simulink model "ManeuverPlanning"  (R2020b)
settings: Solver=FixedStepAuto  StartTime=0.0  StopTime=15  FixedStep=Ts/2  RelTol=1e-3
values from neighbouring files (symbols this model uses):
  Ts = 0.01    [prepare_simulation.m]
undefined symbols (not defined in the file or in its folder): constraints, dimensionsEgo, dimensionsLead, ego, laneWidth, lateral, other, road, roadTrajectory, uncertainty, v_max, v_min, wheelBaseEgo, wheelBaseLead, xEgo_0, yawEgo_0, yEgo_0
libraries: sim3dautolib x3, mpcadaslib x2, vrlib x2, simulink x2, robotalgslib x1, drivingvehiclecontroller x1, pid_lib x1, sim3dlib x1, robotmobilelib x1
(part 1 of 2)
settings Model: Creator=Mustafa  LastModifiedBy=mustafa
settings SFSimCC: CustomCodeUndefinedFunction=UseInterfaceOnly

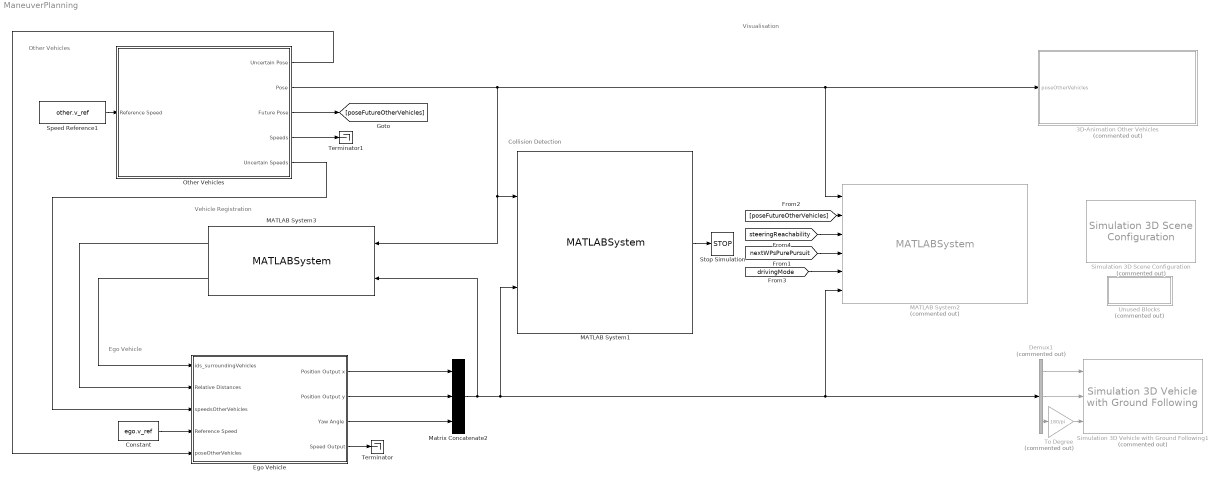
== system ManeuverPlanning ==
  note: Vehicle Registration
  note: Collision Detection
  note: Visualisation
  note: Ego Vehicle
  note: Other Vehicles
  3D-Animation Other Vehicles : Subsystem  Commented=on
  Constant : Constant  Value=ego.v_ref
  Demux1 : Demux  Commented=on  Outputs=3
  Ego Vehicle : Subsystem  mask{Speed=ego.v_0}
      mask prompts: Speed "Initial Speed"
      mask TypeOptions Speed: Initial Speed/Value
  MATLAB System1 : MATLABSystem  System=CollisionDetection  dimensionsEgo=ego.dimensions  wheelBaseEgo=ego.wheelBase  dimensionsOtherVehicles=other.dimensions  wheelBaseOtherVehicles=other.wheelBase  SimulateUsing=Interpreted execution
      mask Type: CollisionDetection
      mask Display:
      | disp('CollisionDetection');
      | port_label('input',1,'poseOtherVehicles');
      | port_label('input',2,'poseEgo');
      | port_label('output',1,'isCollided');
  MATLAB System2 : MATLABSystem  Commented=on  System=PlotDrivingScenario  dimensionsOtherVehicles=other.dimensions  wheelBaseOtherVehicles=other.wheelBase  dimensionsEgo=ego.dimensions  wheelBaseEgo=ego.wheelBase  LaneWidth=road.laneWidth  RoadTrajectory=road.trajectory  spaceDiscretisation=spaceDiscretisation  SimulateUsing=Interpreted execution
      mask Type: PlotDrivingScenario
      mask Display:
      | disp('PlotDrivingScenario');
      | port_label('input',1,'poseOtherVehicles');
      | port_label('input',2,'poseOtherVehiclesFuture');
      | port_label('input',3,'egoReachability');
      | port_label('input',4,'nextWPsPurePursuit');
      | port_label('input',5,'currentDrivingMode');
      | port_label('input',6,'poseEgo');
  MATLAB System3 : MATLABSystem  System=RegisterVehicles  LaneWidth=road.laneWidth  RoadTrajectory=road.trajectory  SimulateUsing=Interpreted execution
      mask Type: RegisterVehicles
      mask Display:
      | disp('RegisterVehicles');
      | port_label('input',1,'poseOtherVehicles');
      | port_label('input',2,'poseEgo');
      | port_label('output',1,'distances2Vehicles');
      | port_label('output',2,'ids_surroundingVehicles');
  Matrix Concatenate2 : Concatenate  NumInputs=3  ConcatenateDimension=2
  Other Vehicles : Subsystem  mask{s_0=other.s_0, d=other.d_0, Speed=other.v_0}
      mask prompts: s_0 "Initial s (Frenet)"; d "d (Frenet)"; Speed "Initial Speed"
      mask TypeOptions s_0: Initial Frenet s-coordinate/Value
      mask TypeOptions d: Frenet d-coordinate/Value
      mask TypeOptions Speed: Initial Speed/Value
  Simulation 3D Scene Configuration : sim3dlib/Simulation 3D Scene Configuration  Priority=0  Commented=on  ProjectFormat=Default Scenes  SceneDesc=Straight road  ProjectName=VehicleSimulation.exe  ScenePath=/Game/Maps/HwStrght  vehTagList={'Scene Origin';'SimulinkVehicle1';'SimulinkVehicle2';'SimulinkVehicleEgo'}  vehTag=SimulinkVehicleEgo  OpVisEn=off  Ts=0.1  EnableWindow=on  sensorTag=MainCamera1  sensorId=1  sensorName=MainCamera1  mountLoc=Origin  offsetFlag=off  tmountOffset=[0, 0, 0]  rmountOffset=[0, 0, 0]  HorizontalResolution=1280  VerticalResolution=720  HorizontalFOV=60  mountPoint=[0 0 0]  mountOrientation=[0 0 0]  aMode=3  ID=1
      settings: SourceProductBaseCode=DR,UV,VE
  Simulation 3D Vehicle with Ground Following1 : sim3dautolib/Simulation 3D Vehicle with Ground Following  Priority=-1  Commented=on  PassVehMesh=Muscle car  VehColor=Red  InitialPos=[ego.x_0, ego.y_0, ego.yaw_0]  InitialRot=[0, 0, 0]  ActorName=SimulinkVehicleEgo  SampleTime=0.1  ActorType=SimulinkVehicle  ID=C  aMode=3  ActorTag=SimulinkVehicleEgo  CoordinateScheme=ISO  TransformOutportEnabled=off
      settings: SourceProductBaseCode=DR,UV,VE
  Speed Reference1 : Constant  Value=other.v_ref
  Stop Simulation : Stop
  Terminator : Terminator
  Terminator1 : Terminator
  To Degree : Gain  Commented=on  Gain=180/pi
  Unused Blocks : Subsystem  Commented=on
  wires:
  Ego Vehicle/1(Position Output x) -> Matrix Concatenate2/1
  Ego Vehicle/4(Speed Output) -> Terminator/1
  Ego Vehicle/2(Position Output y) -> Matrix Concatenate2/2
  Ego Vehicle/3(Yaw Angle) -> Matrix Concatenate2/3
  Matrix Concatenate2/1 -> MATLAB System3/2, MATLAB System1/2, MATLAB System2/6, Demux1/1
  Demux1/1 -> Simulation 3D Vehicle with Ground Following1/1
  Demux1/2 -> Simulation 3D Vehicle with Ground Following1/2
  Demux1/3 -> To Degree/1
  To Degree/1 -> Simulation 3D Vehicle with Ground Following1/3
  MATLAB System1/1 -> Stop Simulation/1
  Other Vehicles/2(Pose) -> MATLAB System1/1, MATLAB System3/1, MATLAB System2/1, 3D-Animation Other Vehicles/1(poseOtherVehicles)
  Constant/1 -> Ego Vehicle/4(Reference Speed)
  MATLAB System3/2 -> Ego Vehicle/1(ids_surroundingVehicles)
  MATLAB System3/1 -> Ego Vehicle/2(Relative Distances)
  [poseFutureOtherVehicles] -> MATLAB System2/2
  Other Vehicles/3(Future Pose) -> [poseFutureOtherVehicles]
  [steeringReachability] -> MATLAB System2/3
  [nextWPsPurePursuit] -> MATLAB System2/4
  [drivingMode] -> MATLAB System2/5
  Speed Reference1/1 -> Other Vehicles/1(Reference Speed)
  Other Vehicles/1(Uncertain Pose) -> Ego Vehicle/5(poseOtherVehicles)
  Other Vehicles/5(Uncertain Speeds) -> Ego Vehicle/3(speedsOtherVehicles)
  Other Vehicles/4(Speeds) -> Terminator1/1

== system ManeuverPlanning/3D-Animation Other Vehicles ==
  poseOtherVehicles : Inport
  Demux : Demux  Outputs=3
  Demux1 : Demux  Outputs=3
  Selector : Selector  NumberOfDimensions=2  InputPortWidth=3  IndexOptions=Select all,Index vector (dialog)  Indices=[1 3],1  OutputSizes=1,1
  Selector1 : Selector  NumberOfDimensions=2  InputPortWidth=3  IndexOptions=Select all,Index vector (dialog)  Indices=[1 3],2  OutputSizes=1,1
  Simulation 3D Vehicle with Ground Following : sim3dautolib/Simulation 3D Vehicle with Ground Following  Priority=-1  PassVehMesh=Small pickup truck  VehColor=Blue  InitialPos=[other.x_0(1), other.y_0(1), other.yaw_0(1)]  InitialRot=[0, 0, 0]  ActorName=SimulinkVehicle1  SampleTime=0.1  ActorType=SimulinkVehicle  ID=1  aMode=3  ActorTag=SimulinkVehicle1  CoordinateScheme=ISO  TransformOutportEnabled=off
      settings: SourceProductBaseCode=DR,UV,VE
  Simulation 3D Vehicle with Ground Following1 : sim3dautolib/Simulation 3D Vehicle with Ground Following  Priority=-1  PassVehMesh=Sedan  VehColor=Blue  InitialPos=[other.x_0(2), other.y_0(2), other.yaw_0(2)]  InitialRot=[0, 0, 0]  ActorName=SimulinkVehicle2  SampleTime=0.1  ActorType=SimulinkVehicle  ID=2  aMode=3  ActorTag=SimulinkVehicle2  CoordinateScheme=ISO  TransformOutportEnabled=off
      settings: SourceProductBaseCode=DR,UV,VE
  To Degree1 : Gain  Gain=180/pi
  To Degree2 : Gain  Gain=180/pi
  wires:
  Demux/2 -> Simulation 3D Vehicle with Ground Following/2
  Demux/1 -> Simulation 3D Vehicle with Ground Following/1
  Demux/3 -> To Degree1/1
  To Degree1/1 -> Simulation 3D Vehicle with Ground Following/3
  To Degree2/1 -> Simulation 3D Vehicle with Ground Following1/3
  Demux1/1 -> Simulation 3D Vehicle with Ground Following1/1
  Demux1/3 -> To Degree2/1
  Demux1/2 -> Simulation 3D Vehicle with Ground Following1/2
  poseOtherVehicles/1 -> Selector/1, Selector1/1
  Selector/1 -> Demux/1
  Selector1/1 -> Demux1/1

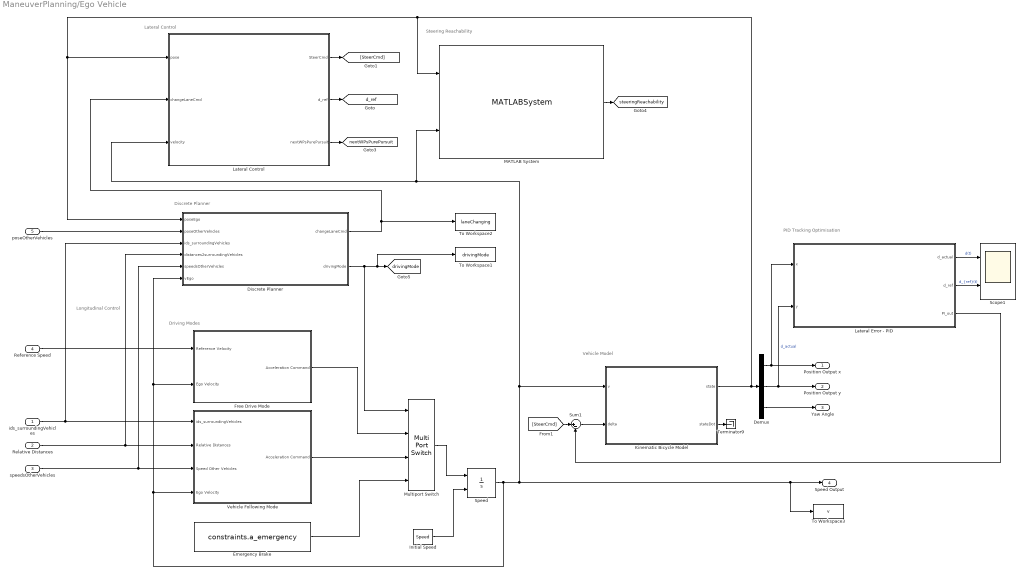
== system ManeuverPlanning/Ego Vehicle ==
  note: PID Tracking Optimisation
  note: Vehicle Model
  note: Discrete Planner
  note: Driving Modes
  note: Longitudinal Control
  note: Lateral Control
  note: Steering Reachability
  ids_surroundingVehicles : Inport
  Relative Distances : Inport  Port=2
  speedsOtherVehicles : Inport  Port=3
  Reference Speed : Inport  Port=4
  poseOtherVehicles : Inport  Port=5
  Demux : Demux  Outputs=3
  Discrete Planner : Subsystem  Variant=on  VariantControlMode=label  LabelModeActiveChoice=POMDP  mask{modePlanner=POMDP}
      mask prompts: modePlanner "Planner Mode:"
      mask TypeOptions modePlanner: MANUAL | FORMAL | NEWPLANNER | POMDP
      mask Callback modePlanner: set_param(gcb,'OverrideUsingVariant',get_param(gcb,'modePlanner'));
  Emergency Brake : Constant  Value=constraints.a_emergency
  Free Drive Mode : Subsystem
  Initial Speed : Constant  Value=Speed
  Kinematic Bicycle Model : Subsystem  mask{L=ego.wheelBase, v_min=constraints.v_min, v_max=constraints.v_max, delta_min=-constraints.steerAngle_max, delta_max=constraints.steerAngle_max, x_0=ego.x_0, y_0=ego.y_0, theta_0=ego.yaw_0}
      mask prompts: L "Wheel base (m):"; v_min "Minimum velocity (m/s):"; v_max "Maximum velocity (m/s):"; delta_min "Minimum steering angle (rad):"; delta_max "Maximum steering angle (rad):"; x_0 "Initial x (m):"; y_0 "Initial y (m):"; theta_0 "Initial orientation (rad):"
      mask TypeOptions L: wheel base/Value
      mask TypeOptions v_min: limit velocity/LowerLimit
      mask TypeOptions v_max: limit velocity/UpperLimit
      mask TypeOptions delta_min: limit steering angle/LowerLimit
      mask TypeOptions delta_max: limit steering angle/UpperLimit
      mask TypeOptions x_0: x_0/Value
      mask TypeOptions y_0: y_0/Value
      mask TypeOptions theta_0: theta_0/Value
  Lateral Control : Subsystem  Variant=on  VariantControlMode=label  LabelModeActiveChoice=STANLEY  mask{modeLateral=STANLEY}
      mask prompts: modeLateral "Lateral Mode:"
      mask TypeOptions modeLateral: PURE_PURSUIT | STANLEY
      mask Callback modeLateral: set_param(gcb,'OverrideUsingVariant',get_param(gcb,'modeLateral'))
  Lateral Error - PID : Subsystem
  MATLAB System : MATLABSystem  System=SteeringReachability  minimumAcceleration=constraints.a_min  maximumAcceleration=constraints.a_max  emergencyAcceleration=constraints.a_emergency  maximumVelocity=constraints.v_max  RoadTrajectory=road.trajectory  wheelBase=ego.wheelBase  steerAngle_max=constraints.steerAngle_max  timeHorizon=trajectoryGeneration.timeHorizon  Ts=Ts  SimulateUsing=Interpreted execution
      mask Type: SteeringReachability
      mask Display:
      | disp('SteeringReachability');
      | port_label('input',1,'pose');
      | port_label('input',2,'v');
      | port_label('output',1,'steeringReachability');
  Multiport Switch : MultiPortSwitch
  Scope1 : Scope  NumInputPorts=2
  Speed : Integrator  InitialConditionSource=external  LimitOutput=on  UpperSaturationLimit=constraints.v_max  LowerSaturationLimit=constraints.v_min
  Sum1 : Sum  Inputs=|+-
  Terminator9 : Terminator
  To Workspace1 : ToWorkspace  VariableName=drivingMode  SampleTime=-1
      settings: Save2DSignal=2-D array (concatenate along first dimension)
  To Workspace2 : ToWorkspace  VariableName=laneChanging  SampleTime=-1
      settings: Save2DSignal=2-D array (concatenate along first dimension)
  To Workspace3 : ToWorkspace  VariableName=v  SampleTime=-1
      settings: Save2DSignal=2-D array (concatenate along first dimension)
  Vehicle Following Mode : Subsystem
  Position Output x : Outport  VectorParamsAs1DForOutWhenUnconnected=off
  Position Output y : Outport  Port=2  VectorParamsAs1DForOutWhenUnconnected=off
  Yaw Angle : Outport  Port=3  VectorParamsAs1DForOutWhenUnconnected=off
  Speed Output : Outport  Port=4  VectorParamsAs1DForOutWhenUnconnected=off
  tag scope: d_ref=global, drivingMode=global, nextWPsPurePursuit=global, steeringReachability=global
  wires:
  Initial Speed/1 -> Speed/2
  Vehicle Following Mode/1(Acceleration Command) -> Multiport Switch/3
  Multiport Switch/1 -> Speed/1
  Free Drive Mode/1(Acceleration Command) -> Multiport Switch/2
  Emergency Brake/1 -> Multiport Switch/4
  Demux/3 -> Yaw Angle/1
  Kinematic Bicycle Model/2(stateDot) -> Terminator9/1
  Demux/2 -> Position Output y/1, Lateral Error - PID/2(y)  "d_actual"
  Lateral Control/1(SteerCmd) -> [SteerCmd]
  Lateral Control/2(d_ref) -> [d_ref]
  Discrete Planner/1(changeLaneCmd) -> Lateral Control/2(changeLaneCmd), To Workspace2/1
  Speed/1 -> To Workspace3/1, Speed Output/1, Kinematic Bicycle Model/1(v), MATLAB System/2, Lateral Control/3(velocity), Vehicle Following Mode/4(Ego Velocity), Discrete Planner/6(vEgo), Free Drive Mode/2(Ego Velocity)
  Kinematic Bicycle Model/1(state) -> MATLAB System/1, Discrete Planner/1(poseEgo), Lateral Control/1(pose), Demux/1
  Lateral Control/3(nextWPsPurePursuit) -> [nextWPsPurePursuit]
  Sum1/1 -> Kinematic Bicycle Model/2(delta)
  [SteerCmd] -> Sum1/1
  Lateral Error - PID/3(PI_out) -> Sum1/2
  Demux/1 -> Position Output x/1, Lateral Error - PID/1(x)
  Lateral Error - PID/1(d_actual) -> Scope1/1  "d(t)"
  Lateral Error - PID/2(d_ref) -> Scope1/2  "d_{ref}(t)"
  Reference Speed/1 -> Free Drive Mode/1(Reference Velocity)
  Relative Distances/1 -> Discrete Planner/4(distances2surroundingVehicles), Vehicle Following Mode/2(Relative Distances)
  speedsOtherVehicles/1 -> Discrete Planner/5(speedsOtherVehicles), Vehicle Following Mode/3(Speed Other Vehicles)
  Discrete Planner/2(drivingMode) -> Multiport Switch/1, To Workspace1/1, [drivingMode]
  ids_surroundingVehicles/1 -> Discrete Planner/3(ids_surroundingVehicles), Vehicle Following Mode/1(ids_surroundingVehicles)
  MATLAB System/1 -> [steeringReachability]
  poseOtherVehicles/1 -> Discrete Planner/2(poseOtherVehicles)

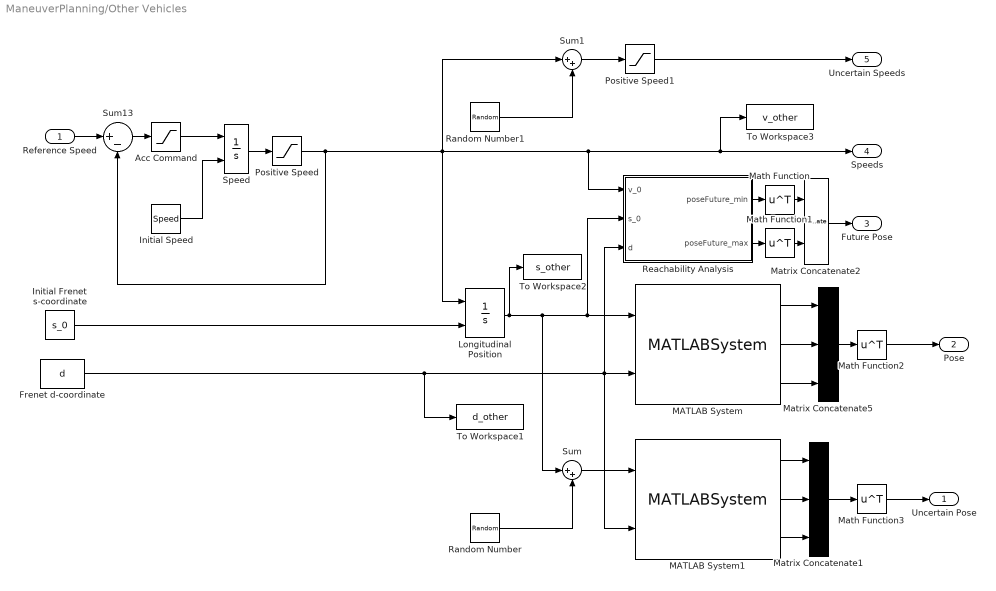
== system ManeuverPlanning/Other Vehicles ==
  Reference Speed : Inport
  Acc Command : Saturate  UpperLimit=constraints.a_max  LowerLimit=constraints.a_min
  Frenet d-coordinate : Constant  Value=d
  Initial Frenet s-coordinate : Constant  Value=s_0
  Initial Speed : Constant  Value=Speed
  Longitudinal Position : Integrator  InitialConditionSource=external
  MATLAB System : MATLABSystem  System=Frenet2CartesianSystem  RoadTrajectory=road.trajectory  lengthOut=other.number  SimulateUsing=Interpreted execution
      mask Type: Frenet2CartesianSystem
      mask Display:
      | disp('Frenet2CartesianSystem');
      | port_label('input',1,'s');
      | port_label('input',2,'d');
      | port_label('output',1,'x');
      | port_label('output',2,'y');
      | port_label('output',3,'refOrientation');
  MATLAB System1 : MATLABSystem  System=Frenet2CartesianSystem  RoadTrajectory=road.trajectory  lengthOut=other.number  SimulateUsing=Interpreted execution
      mask Type: Frenet2CartesianSystem
      mask Display:
      | disp('Frenet2CartesianSystem');
      | port_label('input',1,'s');
      | port_label('input',2,'d');
      | port_label('output',1,'x');
      | port_label('output',2,'y');
      | port_label('output',3,'refOrientation');
  Math Function{,1..3} (4 alike) : Math  Operator=transpose  SaturateOnIntegerOverflow=on
  Matrix Concatenate1 : Concatenate  NumInputs=3  Mode=Multidimensional array  ConcatenateDimension=2
  Matrix Concatenate2 : Concatenate  Mode=Multidimensional array
  Matrix Concatenate5 : Concatenate  NumInputs=3  Mode=Multidimensional array  ConcatenateDimension=2
  Positive Speed : Saturate  UpperLimit=constraints.v_max  LowerLimit=constraints.v_min
  Positive Speed1 : Saturate  UpperLimit=constraints.v_max  LowerLimit=constraints.v_min
  Random Number : RandomNumber  Variance=uncertainty.sigmaS^2  SampleTime=Ts
  Random Number1 : RandomNumber  Variance=uncertainty.sigmaV^2  SampleTime=Ts
  Reachability Analysis : Subsystem
  Speed : Integrator  InitialConditionSource=external
  Sum : Sum  Inputs=|++
  Sum1 : Sum  Inputs=|++
  Sum13 : Sum  Inputs=|+-
  To Workspace1 : ToWorkspace  VariableName=d_other  SampleTime=-1
      settings: Save2DSignal=2-D array (concatenate along first dimension)
  To Workspace2 : ToWorkspace  VariableName=s_other  SampleTime=-1
      settings: Save2DSignal=2-D array (concatenate along first dimension)
  To Workspace3 : ToWorkspace  VariableName=v_other  SampleTime=-1
      settings: Save2DSignal=2-D array (concatenate along first dimension)
  Uncertain Pose : Outport  VectorParamsAs1DForOutWhenUnconnected=off
  Pose : Outport  Port=2
  Future Pose : Outport  Port=3
  Speeds : Outport  Port=4  VectorParamsAs1DForOutWhenUnconnected=off
  Uncertain Speeds : Outport  Port=5  VectorParamsAs1DForOutWhenUnconnected=off
  wires:
  Speed/1 -> Positive Speed/1
  Initial Frenet s-coordinate/1 -> Longitudinal Position/2
  Sum13/1 -> Acc Command/1
  Reference Speed/1 -> Sum13/1
  Acc Command/1 -> Speed/1
  Initial Speed/1 -> Speed/2
  Frenet d-coordinate/1 -> To Workspace1/1, MATLAB System1/2, MATLAB System/2, Reachability Analysis/3(d)
  Longitudinal Position/1 -> Sum/1, MATLAB System/1, Reachability Analysis/2(s_0), To Workspace2/1
  Matrix Concatenate2/1 -> Future Pose/1
  Reachability Analysis/1(poseFuture_min) -> Math Function/1
  Math Function/1 -> Matrix Concatenate2/1
  Reachability Analysis/2(poseFuture_max) -> Math Function1/1
  Math Function1/1 -> Matrix Concatenate2/2
  Matrix Concatenate5/1 -> Math Function2/1
  MATLAB System/2 -> Matrix Concatenate5/2
  MATLAB System/1 -> Matrix Concatenate5/1
  MATLAB System/3 -> Matrix Concatenate5/3
  Math Function2/1 -> Pose/1
  Math Function3/1 -> Uncertain Pose/1
  Matrix Concatenate1/1 -> Math Function3/1
  MATLAB System1/3 -> Matrix Concatenate1/3
  MATLAB System1/2 -> Matrix Concatenate1/2
  MATLAB System1/1 -> Matrix Concatenate1/1
  Sum/1 -> MATLAB System1/1
  Random Number/1 -> Sum/2
  Random Number1/1 -> Sum1/2
  Sum1/1 -> Positive Speed1/1
  Positive Speed1/1 -> Uncertain Speeds/1
  Positive Speed/1 -> Sum1/1, To Workspace3/1, Speeds/1, Reachability Analysis/1(v_0), Longitudinal Position/1, Sum13/2

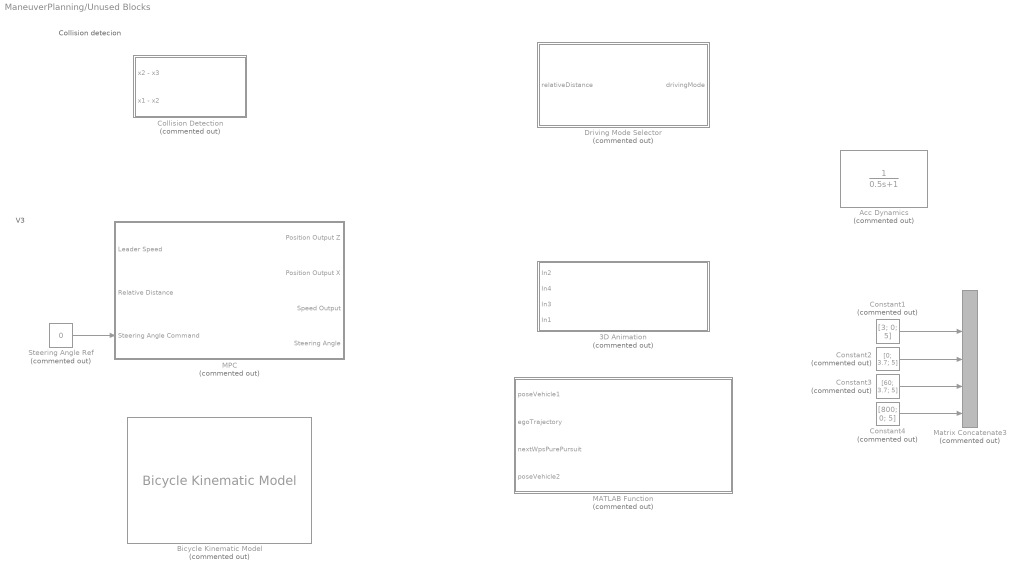
== system ManeuverPlanning/Unused Blocks ==
  note: V3
  note: Collision detecion
  3D Animation : Subsystem  Commented=on
  Acc Dynamics : TransferFcn  Commented=on  Denominator=[0.5 1]
  Bicycle Kinematic Model : robotmobilelib/Bicycle Kinematic Model  Commented=on  VehicleInputs=Vehicle Speed & Steering Angle  WheelBase=wheelBaseEgo  VehicleSpeedRange=[v_min v_max]  MaxSteeringAngle=steerAngle_max  InitialState=[xEgo_0; yEgo_0; yawEgo_0]  SimulateUsing=Interpreted execution
      settings: SourceProductBaseCode=RO
  Collision Detection : Subsystem  Commented=on
  Constant1 : Constant  Commented=on  Value=[3; 0; 5]
  Constant2 : Constant  Commented=on  Value=[0; 3.7; 5]
  Constant3 : Constant  Commented=on  Value=[60; 3.7; 5]
  Constant4 : Constant  Commented=on  Value=[800; 0; 5]
  Driving Mode Selector : Stateflow chart  Commented=on  TreatAsAtomicUnit=on
  MATLAB Function : MATLAB Function  Commented=on  TreatAsAtomicUnit=on  SystemSampleTime=0.1  mask{dimensionsVehicle1=dimensionsLead, wheelBaseVehicle1=wheelBaseLead, dimensionsVehicle2=dimensionsEgo, wheelBaseVehicle2=wheelBaseEgo, LaneWidth=laneWidth, roadTrajectory=roadTrajectory}
      mask prompts: dimensionsVehicle1 "Dimensions (length, width) vehicle 1"; wheelBaseVehicle1 "Wheel base vehicle 1"; dimensionsVehicle2 "Dimensions (length, width) vehicle 2"; wheelBaseVehicle2 "Wheel base vehicle 2"; LaneWidth "Lane width"; roadTrajectory "Road trajectory according to MOBATSim map format"
      mask init:
      | close all;
      | figure('units','normalized','outerposition',[0 0 1 1]);
      | grid on
      | axis equal
      | hold on
  MPC : Subsystem  Commented=on  mask{Pos=20, Speed=25}
      mask prompts: Pos "Initial Position"; Speed "Initial Speed"
      mask TypeOptions Pos: Initial Position Z/Value
      mask TypeOptions Speed: Initial Speed/Value
  Matrix Concatenate3 : Concatenate  Commented=on  NumInputs=5  Mode=Multidimensional array  ConcatenateDimension=2
  Steering Angle Ref : Constant  Commented=on  Value=0
  wires:
  Steering Angle Ref/1 -> MPC/3(Steering Angle Command)
  Constant3/1 -> Matrix Concatenate3/4
  Constant4/1 -> Matrix Concatenate3/5
  Constant2/1 -> Matrix Concatenate3/3
  Constant1/1 -> Matrix Concatenate3/2

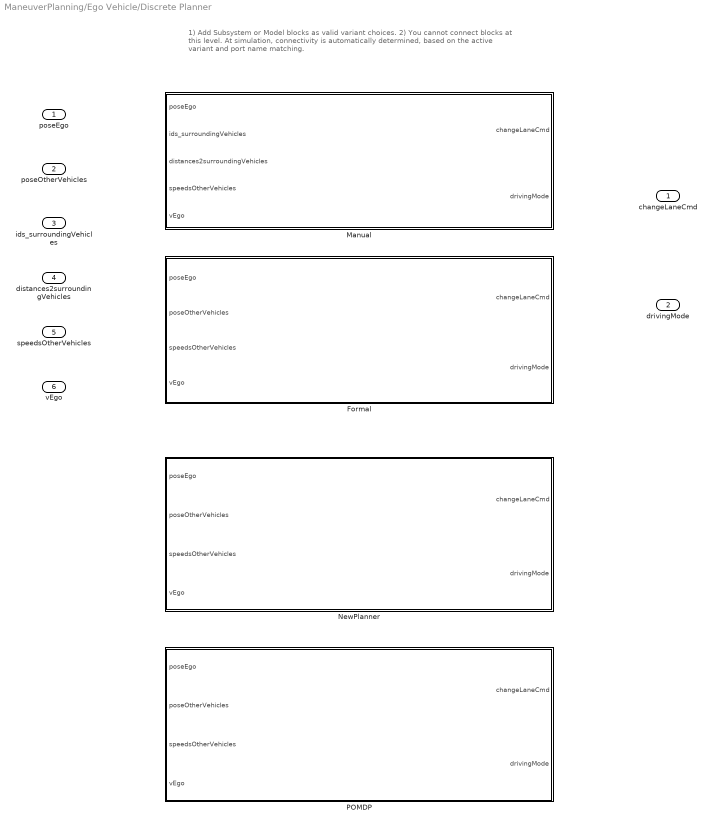
== system ManeuverPlanning/Ego Vehicle/Discrete Planner ==
  note: 1) Add Subsystem or Model blocks as valid variant choices.
      | 2) You cannot connect blocks at this level. At simulation, connectivity is automatically
      | determined, based on the active variant and port name matching.
  poseEgo : Inport
  poseOtherVehicles : Inport  Port=2
  ids_surroundingVehicles : Inport  Port=3
  distances2surroundingVehicles : Inport  Port=4
  speedsOtherVehicles : Inport  Port=5
  vEgo : Inport  Port=6
  Formal : Subsystem  VariantControl=FORMAL
  Manual : Subsystem  VariantControl=MANUAL
  NewPlanner : Subsystem  VariantControl=NEWPLANNER
  POMDP : Subsystem  VariantControl=POMDP
  changeLaneCmd : Outport
  drivingMode : Outport  Port=2

== system ManeuverPlanning/Ego Vehicle/Free Drive Mode ==
  Reference Velocity : Inport
  Ego Velocity : Inport  Port=2
  Acc Command : Saturate  UpperLimit=constraints.a_max  LowerLimit=constraints.a_min
  Sum13 : Sum  Inputs=|+-
  Acceleration Command : Outport
  wires:
  Sum13/1 -> Acc Command/1
  Acc Command/1 -> Acceleration Command/1
  Reference Velocity/1 -> Sum13/1
  Ego Velocity/1 -> Sum13/2

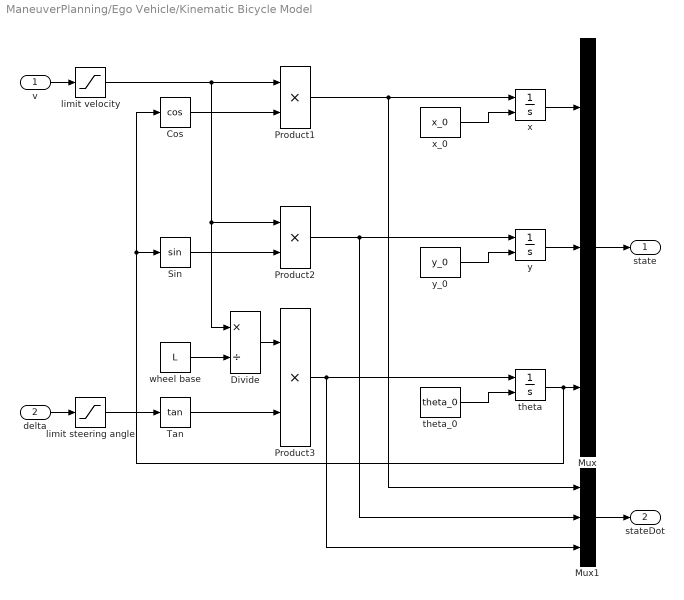
== system ManeuverPlanning/Ego Vehicle/Kinematic Bicycle Model ==
  v : Inport
  delta : Inport  Port=2
  Cos : Trigonometry  Operator=cos
  Divide : Product  Inputs=*/
  Mux : Mux  Inputs=3
  Mux1 : Mux  Inputs=3
  Product1 : Product
  Product2 : Product
  Product3 : Product
  Sin : Trigonometry
  Tan : Trigonometry  Operator=tan
  limit steering angle : Saturate  UpperLimit=delta_max  LowerLimit=delta_min
  limit velocity : Saturate  UpperLimit=v_max  LowerLimit=v_min
  theta : Integrator  InitialConditionSource=external
  theta_0 : Constant  Value=theta_0
  wheel base : Constant  Value=L
  x : Integrator  InitialConditionSource=external
  x_0 : Constant  Value=x_0
  y : Integrator  InitialConditionSource=external
  y_0 : Constant  Value=y_0
  state : Outport
  stateDot : Outport  Port=2
  wires:
  Mux/1 -> state/1
  Mux1/1 -> stateDot/1
  v/1 -> limit velocity/1
  Sin/1 -> Product2/2
  Cos/1 -> Product1/2
  Tan/1 -> Product3/2
  Product1/1 -> Mux1/1, x/1
  Product2/1 -> Mux1/2, y/1
  Product3/1 -> Mux1/3, theta/1
  theta/1 -> Cos/1, Sin/1, Mux/3
  x/1 -> Mux/1
  y/1 -> Mux/2
  Divide/1 -> Product3/1
  wheel base/1 -> Divide/2
  limit velocity/1 -> Product1/1, Divide/1, Product2/1
  x_0/1 -> x/2
  y_0/1 -> y/2
  theta_0/1 -> theta/2
  delta/1 -> limit steering angle/1
  limit steering angle/1 -> Tan/1

== system ManeuverPlanning/Ego Vehicle/Lateral Control ==
  note: 1) Add Subsystem or Model blocks as valid variant choices.
      | 2) You cannot connect blocks at this level. At simulation, connectivity is automatically
      | determined, based on the active variant and port name matching.
  pose : Inport
  changeLaneCmd : Inport  Port=2
  velocity : Inport  Port=3
  Pure Pursuit : Subsystem  VariantControl=PURE_PURSUIT
  Stanley : Subsystem  VariantControl=STANLEY
  SteerCmd : Outport
  d_ref : Outport  Port=2
  nextWPsPurePursuit : Outport  Port=3

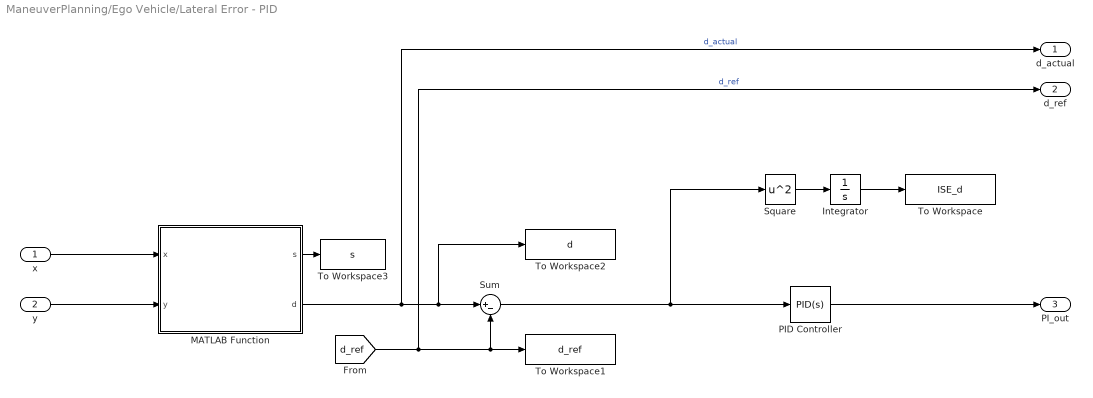
== system ManeuverPlanning/Ego Vehicle/Lateral Error - PID ==
  x : Inport
  y : Inport  Port=2
  Integrator : Integrator
  MATLAB Function : MATLAB Function  TreatAsAtomicUnit=on  mask{currentTrajectory=road.trajectory}
      mask prompts: currentTrajectory "Road trajectory"
  PID Controller : pid_lib/PID Controller  Controller=PID  Form=Parallel  TimeDomain=Continuous-time  UseExternalTs=off  SampleTime=-1  IntegratorMethod=Forward Euler  FilterMethod=Forward Euler  ControllerParametersSource=internal  P=lateral.Kp  I=lateral.Ki  D=lateral.Kd  UseFilter=on  N=100  TunerSelectOption=Transfer Function Based (PID Tuner App)  InitialConditionSource=internal  InitialConditionForIntegrator=0  InitialConditionForFilter=0  DifferentiatorICPrevScaledInput=0  ExternalReset=none  TrackingMode=off  Kt=1  LimitOutput=off  SatLimitsSource=internal  UpperSaturationLimit=inf  LowerSaturationLimit=-inf  LinearizeAsGain=on  AntiWindupMode=none  Kb=1  POutMin=[]  POutMax=[]  IOutMin=[]  IOutMax=[]  DOutMin=[]  DOutMax=[]  NOutMin=[]  NOutMax=[]  SumOutMin=[]  SumOutMax=[]  SaturationOutMin=[]  SaturationOutMax=[]  PParamMin=[]  PParamMax=[]  IParamMin=[]  IParamMax=[]  DParamMin=[]  DParamMax=[]  NParamMin=[]  NParamMax=[]  KbParamMin=[]  KbParamMax=[]  KtParamMin=[]  KtParamMax=[]  KbOutMin=[]  KbOutMax=[]  KtOutMin=[]  KtOutMax=[]  IntegratorOutMin=[]  IntegratorOutMax=[]  FilterOutMin=[]  FilterOutMax=[]  SumI1OutMin=[]  SumI1OutMax=[]  SumI2OutMin=[]  SumI2OutMax=[]  SumI3OutMin=[]  SumI3OutMax=[]  SumI4OutMin=[]  SumI4OutMax=[]  SumDOutMin=[]  SumDOutMax=[]  DifferentiatorOutMin=[]  DifferentiatorOutMax=[]  FilterDiffOutCoefMin=[]  FilterDiffOutCoefMax=[]  ReciprocalOutMin=[]  ReciprocalOutMax=[]  SumDenOutMin=[]  SumDenOutMax=[]  SumNumOutMin=[]  SumNumOutMax=[]  DivideOutMin=[]  DivideOutMax=[]  UdiffTsProdOutMin=[]  UdiffTsProdOutMax=[]  NTsProdOutMin=[]  NTsProdOutMax=[]  UintegralTsProdOutMin=[]  UintegralTsProdOutMax=[]  UngainTsProdOutMin=[]  UngainTsProdOutMax=[]  IntegratorContinuousStateAttributes=''  IntegratorStateMustResolveToSignalObject=off  IntegratorRTWStateStorageClass=Auto  FilterContinuousStateAttributes=''  FilterStateMustResolveToSignalObject=off  FilterRTWStateStorageClass=Auto  ParallelPVariant=InternalParameters  IdealPVariant=Disabled  IVariant=InternalParameters  DVariant=InternalParameters  IntegratorVariant=Continuous  SatVariant=Disabled  AWVariant=Passthrough  PCopyVariant=Disabled  TRVariant=Disabled  FdbkBlocksVariant=Forward  IdealPFdbkVariant=Disabled  SatFdbkVariant=Disabled  DerivativeFilterVariant=ContFilter  NVariant=InternalParameters  NCopyVariant=Disabled  FilterICVariant=InternalICsFilter  IntegratorICVariant=InternalICs  ExternalResetVariant=Disabled  TRSumVariant=Passthrough  SumFdbkVariant=Disabled  SumVariant=Sum_PID  TsampFilterVariant=InternalTs  TsampNgainVariant=Passthrough  TsampIntegralVariant=Passthrough  ExternalSaturationOutDataTypeStr=Inherit: Same as second input
  Square : Math  Operator=square  SaturateOnIntegerOverflow=on
  Sum : Sum  Inputs=|+-
  To Workspace : ToWorkspace  VariableName=ISE_d  SampleTime=-1
      settings: Save2DSignal=2-D array (concatenate along first dimension)
  To Workspace1 : ToWorkspace  VariableName=d_ref  SampleTime=-1
      settings: Save2DSignal=2-D array (concatenate along first dimension)
  To Workspace2 : ToWorkspace  VariableName=d  SampleTime=-1
      settings: Save2DSignal=2-D array (concatenate along first dimension)
  To Workspace3 : ToWorkspace  VariableName=s  SampleTime=-1
      settings: Save2DSignal=2-D array (concatenate along first dimension)
  d_actual : Outport
  d_ref : Outport  Port=2
  PI_out : Outport  Port=3
  wires:
  Sum/1 -> PID Controller/1, Square/1
  MATLAB Function/1(s) -> To Workspace3/1
  Integrator/1 -> To Workspace/1
  MATLAB Function/2(d) -> d_actual/1, To Workspace2/1, Sum/1  "d_actual"
  [d_ref] -> d_ref/1, To Workspace1/1, Sum/2  "d_ref"
  Square/1 -> Integrator/1
  y/1 -> MATLAB Function/2(y)
  x/1 -> MATLAB Function/1(x)
  PID Controller/1 -> PI_out/1

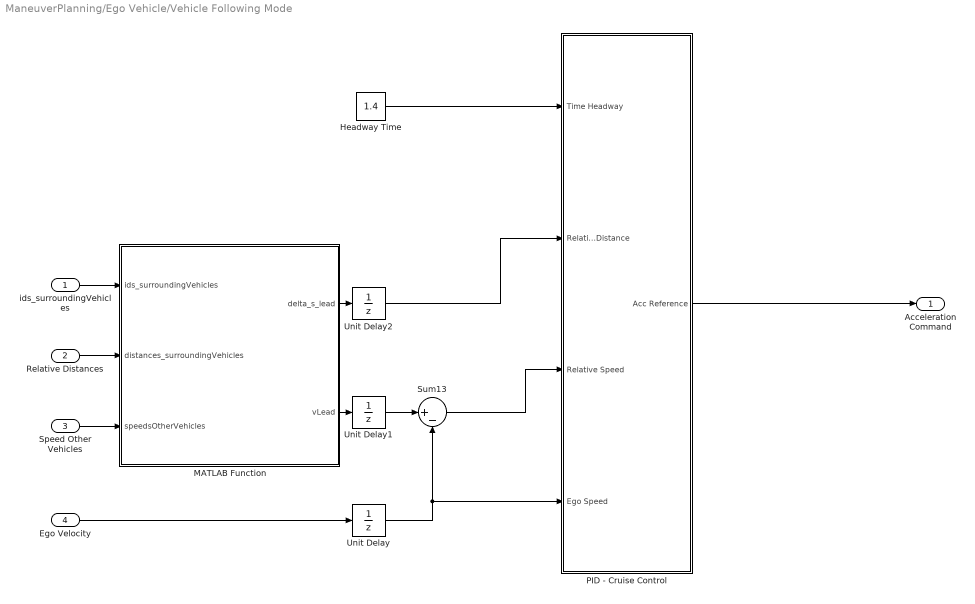
== system ManeuverPlanning/Ego Vehicle/Vehicle Following Mode ==
  ids_surroundingVehicles : Inport
  Relative Distances : Inport  Port=2
  Speed Other Vehicles : Inport  Port=3
  Ego Velocity : Inport  Port=4
  Headway Time : Constant  Value=1.4
  MATLAB Function : MATLAB Function  TreatAsAtomicUnit=on
  PID - Cruise Control : Subsystem
  Sum13 : Sum  Inputs=|+-
  Unit Delay : UnitDelay  SampleTime=-1  HasFrameUpgradeWarning=on
  Unit Delay1 : UnitDelay  SampleTime=-1  HasFrameUpgradeWarning=on
  Unit Delay2 : UnitDelay  SampleTime=-1  HasFrameUpgradeWarning=on
  Acceleration Command : Outport
  wires:
  Headway Time/1 -> PID - Cruise Control/1(Time Headway)
  Sum13/1 -> PID - Cruise Control/3(Relative Speed)
  PID - Cruise Control/1(Acc Reference) -> Acceleration Command/1
  Unit Delay/1 -> Sum13/2, PID - Cruise Control/4(Ego Speed)
  Unit Delay1/1 -> Sum13/1
  Unit Delay2/1 -> PID - Cruise Control/2(Relative Distance)
  MATLAB Function/1(delta_s_lead) -> Unit Delay2/1
  Ego Velocity/1 -> Unit Delay/1
  MATLAB Function/2(vLead) -> Unit Delay1/1
  Speed Other Vehicles/1 -> MATLAB Function/3(speedsOtherVehicles)
  ids_surroundingVehicles/1 -> MATLAB Function/1(ids_surroundingVehicles)
  Relative Distances/1 -> MATLAB Function/2(distances_surroundingVehicles)

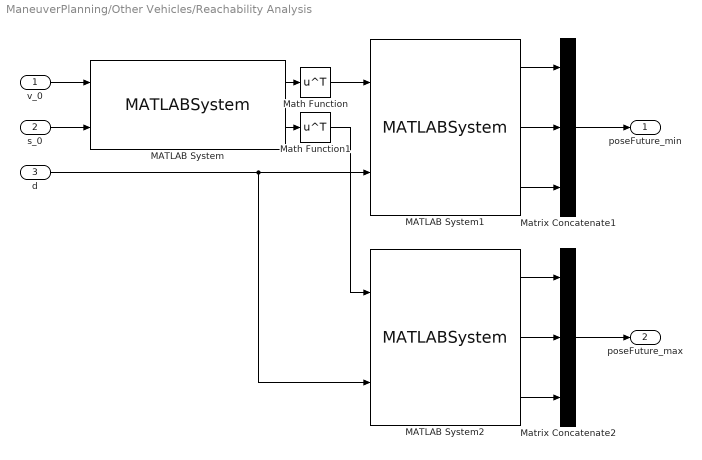
== system ManeuverPlanning/Other Vehicles/Reachability Analysis ==
  v_0 : Inport
  s_0 : Inport  Port=2
  d : Inport  Port=3
  MATLAB System : MATLABSystem  System=LongitudinalReachability  lengthOut=other.number  minimumAcceleration=constraints.a_min  maximumAcceleration=constraints.a_max  emergencyAcceleration=constraints.a_emergency  maximumVelocity=constraints.v_max  RoadTrajectory=road.trajectory  wheelBase=other.wheelBase(1)  steerAngle_max=constraints.steerAngle_max  timeHorizon=trajectoryGeneration.timeHorizon  Ts=Ts  SimulateUsing=Interpreted execution
      mask Type: LongitudinalReachability
      mask Display:
      | disp('LongitudinalReachability');
      | port_label('input',1,'v_0');
      | port_label('input',2,'s_0');
      | port_label('output',1,'sFuture_min');
      | port_label('output',2,'sFuture_max');
  MATLAB System1 : MATLABSystem  System=Frenet2CartesianSystem  RoadTrajectory=road.trajectory  lengthOut=other.number  SimulateUsing=Interpreted execution
      mask Type: Frenet2CartesianSystem
      mask Display:
      | disp('Frenet2CartesianSystem');
      | port_label('input',1,'s');
      | port_label('input',2,'d');
      | port_label('output',1,'x');
      | port_label('output',2,'y');
      | port_label('output',3,'refOrientation');
  MATLAB System2 : MATLABSystem  System=Frenet2CartesianSystem  RoadTrajectory=road.trajectory  lengthOut=other.number  SimulateUsing=Interpreted execution
      mask Type: Frenet2CartesianSystem
      mask Display:
      | disp('Frenet2CartesianSystem');
      | port_label('input',1,'s');
      | port_label('input',2,'d');
      | port_label('output',1,'x');
      | port_label('output',2,'y');
      | port_label('output',3,'refOrientation');
  Math Function : Math  Operator=transpose  SaturateOnIntegerOverflow=on
  Math Function1 : Math  Operator=transpose  SaturateOnIntegerOverflow=on
  Matrix Concatenate1 : Concatenate  NumInputs=3  Mode=Multidimensional array  ConcatenateDimension=2
  Matrix Concatenate2 : Concatenate  NumInputs=3  Mode=Multidimensional array  ConcatenateDimension=2
  poseFuture_min : Outport
  poseFuture_max : Outport  Port=2
  wires:
  s_0/1 -> MATLAB System/2
  v_0/1 -> MATLAB System/1
  d/1 -> MATLAB System2/2, MATLAB System1/2
  MATLAB System1/1 -> Matrix Concatenate1/1
  MATLAB System1/2 -> Matrix Concatenate1/2
  MATLAB System1/3 -> Matrix Concatenate1/3
  MATLAB System2/1 -> Matrix Concatenate2/1
  MATLAB System2/2 -> Matrix Concatenate2/2
  MATLAB System2/3 -> Matrix Concatenate2/3
  Matrix Concatenate1/1 -> poseFuture_min/1
  Matrix Concatenate2/1 -> poseFuture_max/1
  MATLAB System/2 -> Math Function1/1
  Math Function1/1 -> MATLAB System2/1
  MATLAB System/1 -> Math Function/1
  Math Function/1 -> MATLAB System1/1

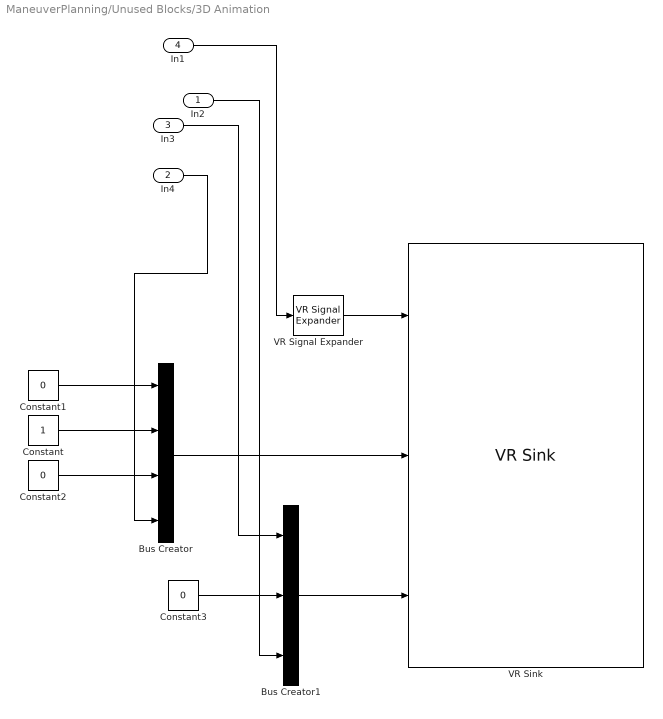
== system ManeuverPlanning/Unused Blocks/3D Animation ==
  In2 : Inport
  In4 : Inport  Port=2
  In3 : Inport  Port=3
  In1 : Inport  Port=4
  Bus Creator : BusCreator  Inputs=4
  Bus Creator1 : BusCreator  Inputs=3
  Constant : Constant
  Constant1 : Constant  Value=0
  Constant2 : Constant  Value=0
  Constant3 : Constant  Value=0
  VR Signal Expander : vrlib/VR Signal Expander  outwidth=3  outidx=[3]
  VR Sink : vrlib/VR Sink  InstantiateOnLoad=on  SampleTime=0.02  ViewEnable=on  RemoteChange=off  RemoteView=off  FieldsWritten=Car_Red.translation.3.1.1.double#Car_Blue.rotation.4.1.1.double#Car_Blue.translation.3.1.1.double  WorldFileName=PlatoonWorld.WRL  AutoView=off  VideoDimensions=[]  AllowVariableSize=off
  wires:
  Constant/1 -> Bus Creator/2
  Constant1/1 -> Bus Creator/1
  Bus Creator1/1 -> VR Sink/3
  In2/1 -> Bus Creator1/3
  Bus Creator/1 -> VR Sink/2
  In4/1 -> Bus Creator/4
  In1/1 -> VR Signal Expander/1
  Constant3/1 -> Bus Creator1/2
  Constant2/1 -> Bus Creator/3
  VR Signal Expander/1 -> VR Sink/1
  In3/1 -> Bus Creator1/1

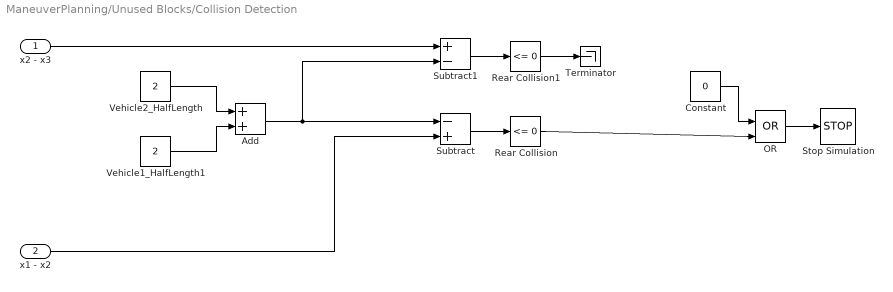
== system ManeuverPlanning/Unused Blocks/Collision Detection ==
  x2 - x3 : Inport
  x1 - x2 : Inport  Port=2
  Add : Sum
  Constant : Constant  Value=0
  OR : Logic  Operator=OR  IconShape=distinctive  AllPortsSameDT=off  OutDataTypeStr=boolean
  Rear Collision : simulink/Logic and Bit Operations/Compare To Constant  relop=<=  const=0  OutDataTypeStr=boolean
  Rear Collision1 : simulink/Logic and Bit Operations/Compare To Constant  relop=<=  const=0  OutDataTypeStr=boolean
  Stop Simulation : Stop
  Subtract : Sum  Inputs=-+
  Subtract1 : Sum  Inputs=+-
  Terminator : Terminator
  Vehicle1_HalfLength1 : Constant  Value=2
  Vehicle2_HalfLength : Constant  Value=2
  wires:
  Vehicle2_HalfLength/1 -> Add/1
  OR/1 -> Stop Simulation/1
  Constant/1 -> OR/1
  Subtract1/1 -> Rear Collision1/1
  Add/1 -> Subtract1/2, Subtract/1
  Rear Collision1/1 -> Terminator/1
  Vehicle1_HalfLength1/1 -> Add/2
  Rear Collision/1 -> OR/2
  Subtract/1 -> Rear Collision/1
  x1 - x2/1 -> Subtract/2
  x2 - x3/1 -> Subtract1/1

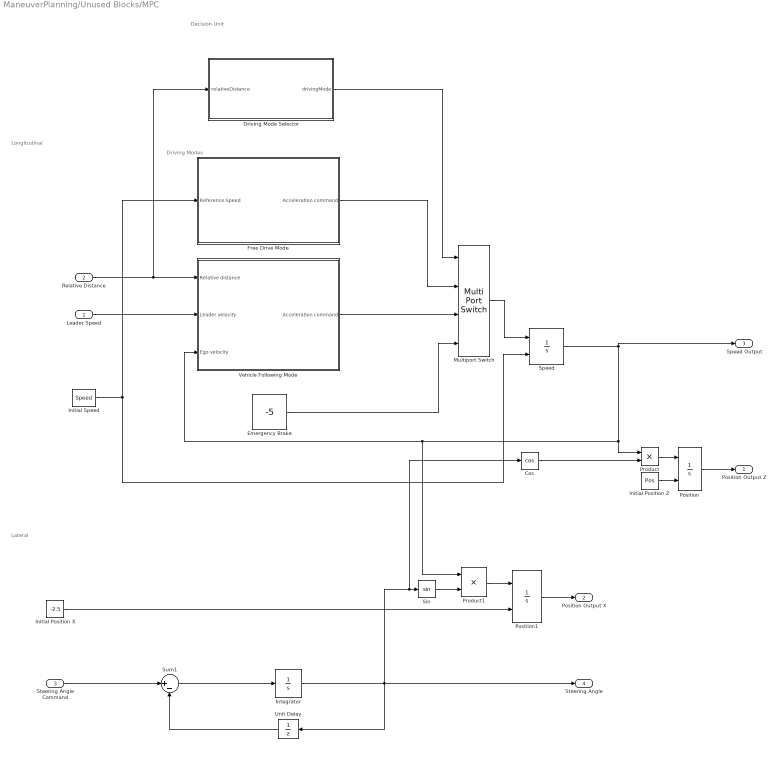
== system ManeuverPlanning/Unused Blocks/MPC ==
  note: Decision Unit
  note: Driving Modes
  note: Longitudinal
  note: Lateral
  Leader Speed : Inport
  Relative Distance : Inport  Port=2
  Steering Angle Command : Inport  Port=3
  Cos : Trigonometry  Operator=cos
  Driving Mode Selector : Stateflow chart  TreatAsAtomicUnit=on
  Emergency Brake : Constant  Value=-5
  Free Drive Mode : Subsystem
  Initial Position X : Constant  Value=-2.5
  Initial Position Z : Constant  Value=Pos
  Initial Speed : Constant  Value=Speed
  Integrator : Integrator
  Multiport Switch : MultiPortSwitch
  Position : Integrator  InitialConditionSource=external
  Position1 : Integrator  InitialConditionSource=external
  Product : Product
  Product1 : Product
  Sin : Trigonometry
  Speed : Integrator  InitialConditionSource=external  LimitOutput=on  LowerSaturationLimit=0
  Sum1 : Sum  Inputs=|+-
  Unit Delay : UnitDelay  SampleTime=-1  HasFrameUpgradeWarning=on
  Vehicle Following Mode : Subsystem
  Position Output Z : Outport  VectorParamsAs1DForOutWhenUnconnected=off
  Position Output X : Outport  Port=2  VectorParamsAs1DForOutWhenUnconnected=off
  Speed Output : Outport  Port=3  VectorParamsAs1DForOutWhenUnconnected=off
  Steering Angle : Outport  Port=4  VectorParamsAs1DForOutWhenUnconnected=off
  wires:
  Position/1 -> Position Output Z/1
  Initial Speed/1 -> Free Drive Mode/1(Reference Speed), Speed/2
  Initial Position Z/1 -> Position/2
  Speed/1 -> Speed Output/1, Vehicle Following Mode/3(Ego velocity), Product1/1, Product/1
  Steering Angle Command/1 -> Sum1/1
  Sum1/1 -> Integrator/1
  Integrator/1 -> Unit Delay/1, Sin/1, Cos/1, Steering Angle/1
  Unit Delay/1 -> Sum1/2
  Initial Position X/1 -> Position1/2
  Cos/1 -> Product/2
  Product/1 -> Position/1
  Sin/1 -> Product1/2
  Product1/1 -> Position1/1
  Position1/1 -> Position Output X/1
  Relative Distance/1 -> Driving Mode Selector/1(relativeDistance), Vehicle Following Mode/1(Relative distance)
  Leader Speed/1 -> Vehicle Following Mode/2(Leader velocity)
  Vehicle Following Mode/1(Acceleration command) -> Multiport Switch/3
  Multiport Switch/1 -> Speed/1
  Free Drive Mode/1(Acceleration command) -> Multiport Switch/2
  Emergency Brake/1 -> Multiport Switch/4
  Driving Mode Selector/1(drivingMode) -> Multiport Switch/1

== system ManeuverPlanning/Ego Vehicle/Discrete Planner/Formal ==
  poseEgo : Inport
  poseOtherVehicles : Inport  Port=2
  speedsOtherVehicles : Inport  Port=3
  vEgo : Inport  Port=4
  MATLAB System1 : MATLABSystem  System=DiscretePlannerFormal  timeHorizon=trajectoryGeneration.timeHorizon  partsTimeHorizon=trajectoryGeneration.partsTimeHorizon  minimumAcceleration=constraints.a_min  maximumAcceleration=constraints.a_max  emergencyAcceleration=constraints.a_emergency  maximumVelocity=constraints.v_max  vOtherVehicles_ref=other.v_ref  wheelBase=ego.wheelBase  steerAngle_max=constraints.steerAngle_max  sigmaS=uncertainty.sigmaS  sigmaV=uncertainty.sigmaV  spaceDiscretisation=spaceDiscretisation  SearchTree=[]  vEgo_ref=ego.v_ref  LaneWidth=road.laneWidth  RoadTrajectory=road.trajectory  Ts=Ts  SimulateUsing=Interpreted execution
      mask Type: DiscretePlannerFormal
      mask Display:
      | disp('DiscretePlannerFormal');
      | port_label('input',1,'poseEgo');
      | port_label('input',2,'poseOtherVehicles');
      | port_label('input',3,'speedsOtherVehicles');
      | port_label('input',4,'vEgo');
      | port_label('output',1,'changeLaneCmd');
      | port_label('output',2,'drivingMode');
  changeLaneCmd : Outport
  drivingMode : Outport  Port=2
  wires:
  poseEgo/1 -> MATLAB System1/1
  poseOtherVehicles/1 -> MATLAB System1/2
  MATLAB System1/1 -> changeLaneCmd/1
  MATLAB System1/2 -> drivingMode/1
  vEgo/1 -> MATLAB System1/4
  speedsOtherVehicles/1 -> MATLAB System1/3

== system ManeuverPlanning/Ego Vehicle/Discrete Planner/Manual ==
  poseEgo : Inport
  ids_surroundingVehicles : Inport  Port=2
  distances2surroundingVehicles : Inport  Port=3
  speedsOtherVehicles : Inport  Port=4
  vEgo : Inport  Port=5
  MATLAB System : MATLABSystem  System=DiscretePlannerManual  vEgo_ref=ego.v_ref  LaneWidth=road.laneWidth  RoadTrajectory=road.trajectory  Ts=Ts  SimulateUsing=Interpreted execution
      mask Type: DiscretePlannerManual
      mask Display:
      | disp('DiscretePlannerManual');
      | port_label('input',1,'poseEgo');
      | port_label('input',2,'ids_surroundingVehicles');
      | port_label('input',3,'distances2surroundingVehicles');
      | port_label('input',4,'speedsOtherVehicles');
      | port_label('input',5,'vEgo');
      | port_label('output',1,'changeLaneCmd');
      | port_label('output',2,'drivingMode');
  changeLaneCmd : Outport
  drivingMode : Outport  Port=2
  wires:
  poseEgo/1 -> MATLAB System/1
  ids_surroundingVehicles/1 -> MATLAB System/2
  distances2surroundingVehicles/1 -> MATLAB System/3
  speedsOtherVehicles/1 -> MATLAB System/4
  vEgo/1 -> MATLAB System/5
  MATLAB System/1 -> changeLaneCmd/1
  MATLAB System/2 -> drivingMode/1

== system ManeuverPlanning/Ego Vehicle/Discrete Planner/NewPlanner ==
  poseEgo : Inport
  poseOtherVehicles : Inport  Port=2
  speedsOtherVehicles : Inport  Port=3
  vEgo : Inport  Port=4
  MATLAB System : MATLABSystem  System=NewPlanner  timeHorizon=trajectoryGeneration.timeHorizon  partsTimeHorizon=trajectoryGeneration.partsTimeHorizon  Ts=Ts  minimumAcceleration=constraints.a_min  maximumAcceleration=constraints.a_max  emergencyAcceleration=constraints.a_emergency  maximumVelocity=constraints.v_max  wheelBase=ego.wheelBase  steerAngle_max=constraints.steerAngle_max  vEgo_ref=ego.v_ref  vOtherVehicles_ref=other.v_ref  sigmaS=uncertainty.sigmaS  sigmaV=uncertainty.sigmaV  LaneWidth=road.laneWidth  RoadTrajectory=road.trajectory  spaceDiscretisation=spaceDiscretisation  SimulateUsing=Interpreted execution
      mask Type: NewPlanner
      mask Display:
      | disp('NewPlanner');
      | port_label('input',1,'poseEgo');
      | port_label('input',2,'poseOtherVehicles');
      | port_label('input',3,'speedsOtherVehicles');
      | port_label('input',4,'vEgo');
      | port_label('output',1,'changeLaneCmd');
      | port_label('output',2,'drivingMode');
  changeLaneCmd : Outport
  drivingMode : Outport  Port=2
  wires:
  vEgo/1 -> MATLAB System/4
  speedsOtherVehicles/1 -> MATLAB System/3
  poseOtherVehicles/1 -> MATLAB System/2
  poseEgo/1 -> MATLAB System/1
  MATLAB System/1 -> changeLaneCmd/1
  MATLAB System/2 -> drivingMode/1

== system ManeuverPlanning/Ego Vehicle/Discrete Planner/POMDP ==
  poseEgo : Inport
  poseOtherVehicles : Inport  Port=2
  speedsOtherVehicles : Inport  Port=3
  vEgo : Inport  Port=4
  MATLAB System : MATLABSystem  System=POMDPPlanner  timeHorizon=trajectoryGeneration.timeHorizon  partsTimeHorizon=trajectoryGeneration.partsTimeHorizon  Ts=Ts  minimumAcceleration=constraints.a_min  maximumAcceleration=constraints.a_max  emergencyAcceleration=constraints.a_emergency  maximumVelocity=constraints.v_max  wheelBase=ego.wheelBase  steerAngle_max=constraints.steerAngle_max  vEgo_ref=ego.v_ref  vOtherVehicles_ref=other.v_ref  sigmaS=uncertainty.sigmaS  sigmaV=uncertainty.sigmaV  LaneWidth=road.laneWidth  RoadTrajectory=road.trajectory  spaceDiscretisation=spaceDiscretisation  SimulateUsing=Interpreted execution
      mask Type: POMDPPlanner
      mask Display:
      | disp('POMDPPlanner');
      | port_label('input',1,'poseEgo');
      | port_label('input',2,'poseOtherVehicles');
      | port_label('input',3,'speedsOtherVehicles');
      | port_label('input',4,'vEgo');
      | port_label('output',1,'changeLaneCmd');
      | port_label('output',2,'drivingMode');
  changeLaneCmd : Outport
  drivingMode : Outport  Port=2
  wires:
  vEgo/1 -> MATLAB System/4
  speedsOtherVehicles/1 -> MATLAB System/3
  poseOtherVehicles/1 -> MATLAB System/2
  poseEgo/1 -> MATLAB System/1
  MATLAB System/1 -> changeLaneCmd/1
  MATLAB System/2 -> drivingMode/1

== system ManeuverPlanning/Ego Vehicle/Lateral Control/Pure Pursuit ==
  pose : Inport
  changeLaneCmd : Inport  Port=2
  velocity : Inport  Port=3
  MATLAB System4 : MATLABSystem  System=PurePursuitWPGenerator  numberWaypoints=lateral.numberWaypoints  maximumAcceleration=constraints.a_max  vEgo_ref=ego.v_ref  LaneWidth=road.laneWidth  RoadTrajectory=road.trajectory  wheelBase=ego.wheelBase  steerAngle_max=constraints.steerAngle_max  timeHorizon=trajectoryGeneration.timeHorizon  Ts=Ts  SimulateUsing=Interpreted execution
      mask Type: PurePursuitWPGenerator
      mask Display:
      | disp('PurePursuitWPGenerator');
      | port_label('input',1,'pose');
      | port_label('input',2,'changeLaneCmd');
      | port_label('input',3,'velocity');
      | port_label('output',1,'nextWPs');
      | port_label('output',2,'d_ref');
  Pure Pursuit1 : robotalgslib/Pure Pursuit  DesiredLinearVelocity=ego.v_ref  MaxAngularVelocity=constraints.angularVelocity_max  LookaheadDistance=lateral.lookAheadDistance  TargetDirPort=on  SimulateUsing=Code generation
  Terminator2 : Terminator
  Terminator3 : Terminator
  Wheel Steering Angle Formulation1 : Subsystem
  SteerCmd : Outport
  d_ref : Outport  Port=2
  nextWPsPurePursuit : Outport  Port=3
  wires:
  Pure Pursuit1/1 -> Terminator2/1
  pose/1 -> Pure Pursuit1/1, MATLAB System4/1
  MATLAB System4/1 -> nextWPsPurePursuit/1, Pure Pursuit1/2
  Pure Pursuit1/3 -> Wheel Steering Angle Formulation1/1(alpha)
  Pure Pursuit1/2 -> Terminator3/1
  MATLAB System4/2 -> d_ref/1
  Wheel Steering Angle Formulation1/1(SteerCmd) -> SteerCmd/1
  velocity/1 -> MATLAB System4/3
  changeLaneCmd/1 -> MATLAB System4/2

== system ManeuverPlanning/Ego Vehicle/Lateral Control/Stanley ==
  pose : Inport
  changeLaneCmd : Inport  Port=2
  velocity : Inport  Port=3
  Constant1 : Constant
  Lateral Controller Stanley1 : drivingvehiclecontroller/Lateral Controller Stanley  ModelType=Kinematic bicycle model  PositionGainF=lateral.forwardMotionGain  PositionGainR=2.5  YawRateGain=0.2  DelayGain=0.2  VehicleMass=1575  Lf=1.2  Lr=1.6  TireStiffness=19000  Wheelbase=ego.wheelBase  MaxSteeringAngle=rad2deg(constraints.steerAngle_max)
      settings: SourceProductBaseCode=DR
  MATLAB System3 : MATLABSystem  System=StanleyPoseGenerator  maximumAcceleration=constraints.a_max  vEgo_ref=ego.v_ref  LaneWidth=road.laneWidth  RoadTrajectory=road.trajectory  wheelBase=ego.wheelBase  steerAngle_max=constraints.steerAngle_max  timeHorizon=trajectoryGeneration.timeHorizon  Ts=Ts  SimulateUsing=Interpreted execution
      mask Type: StanleyPoseGenerator
      mask Display:
      | disp('StanleyPoseGenerator');
      | port_label('input',1,'pose');
      | port_label('input',2,'changeLaneCmd');
      | port_label('input',3,'velocity');
      | port_label('output',1,'d_ref');
      | port_label('output',2,'referencePose');
      | port_label('output',3,'poseOut');
  To radian : Gain  Gain=pi/180
  SteerCmd : Outport
  d_ref : Outport  Port=2
  wires:
  Lateral Controller Stanley1/1 -> To radian/1
  pose/1 -> MATLAB System3/1
  MATLAB System3/1 -> d_ref/1
  Constant1/1 -> Lateral Controller Stanley1/4
  To radian/1 -> SteerCmd/1
  changeLaneCmd/1 -> MATLAB System3/2
  velocity/1 -> MATLAB System3/3, Lateral Controller Stanley1/3
  MATLAB System3/3 -> Lateral Controller Stanley1/2
  MATLAB System3/2 -> Lateral Controller Stanley1/1

== system ManeuverPlanning/Ego Vehicle/Vehicle Following Mode/PID - Cruise Control ==
  Time Headway : Inport
  Relative Distance : Inport  Port=2
  Relative Speed : Inport  Port=3
  Ego Speed : Inport  Port=4
  Adaptive Cruise Control System1 : mpcadaslib/Adaptive Cruise Control System  Commented=on  EgoModel=tf(1,[0.5,1,0])  InitialEgoVelocity=20  DefaultSpacing=10  MaxVelocity=20  MinAcceleration=-3  amin_ext=off  MaxAcceleration=2  amax_ext=off  Ts=0.5  PredictionHorizon=10  ControllerBehavior=0.58999999999999997  suboptimal=off  maxiter=100  datatypeopt=double  optmode=off  trackmode=off
  Constant1 : Constant  Value=20
  Mux : Mux  Inputs=3
  S-Function : S-Function  FunctionName=MPC  SFunctionDeploymentMode=off  EnableBusSupport=off
  Terminator : Terminator
  Terminator1 : Terminator
  Acc Reference : Outport
  wires:
  Ego Speed/1 -> Mux/3
  Time Headway/1 -> Terminator1/1
  Relative Distance/1 -> Mux/1
  Relative Speed/1 -> Mux/2
  Constant1/1 -> Terminator/1
  S-Function/1 -> Acc Reference/1
  Mux/1 -> S-Function/1

== system ManeuverPlanning/Unused Blocks/MPC/Free Drive Mode ==
  Reference Speed : Inport
  Acc Command : Saturate  UpperLimit=2  LowerLimit=-3
  Acc Dynamics : TransferFcn  Denominator=[0.5 1]
  Sum13 : Sum  Inputs=|+-
  Acceleration command : Outport
  wires:
  Sum13/1 -> Acc Command/1
  Acc Dynamics/1 -> Acceleration command/1, Sum13/2
  Reference Speed/1 -> Sum13/1
  Acc Command/1 -> Acc Dynamics/1

== system ManeuverPlanning/Unused Blocks/MPC/Vehicle Following Mode ==
  Relative distance : Inport
  Leader velocity : Inport  Port=2
  Ego velocity : Inport  Port=3
  Acc Dynamics : TransferFcn  Denominator=[0.5 1]
  Adaptive Cruise Control System : mpcadaslib/Adaptive Cruise Control System  EgoModel=tf(1,[0.5,1,0])  InitialEgoVelocity=30  DefaultSpacing=10  MaxVelocity=50  MinAcceleration=-3  amin_ext=off  MaxAcceleration=2  amax_ext=off  Ts=0.5  PredictionHorizon=200  ControllerBehavior=0.590  suboptimal=off  maxiter=100  datatypeopt=double  optmode=off  trackmode=off
  Headway Time : Constant  Value=1.4
  Reference Velocity : Constant  Value=30
  Sum13 : Sum  Inputs=|+-
  Acceleration command : Outport
  wires:
  Leader velocity/1 -> Sum13/1
  Headway Time/1 -> Adaptive Cruise Control System/2
  Reference Velocity/1 -> Adaptive Cruise Control System/1
  Ego velocity/1 -> Adaptive Cruise Control System/3, Sum13/2
  Sum13/1 -> Adaptive Cruise Control System/5
  Relative distance/1 -> Adaptive Cruise Control System/4
  Adaptive Cruise Control System/1 -> Acc Dynamics/1
  Acc Dynamics/1 -> Acceleration command/1

== system ManeuverPlanning/Ego Vehicle/Lateral Control/Pure Pursuit/Wheel Steering Angle Formulation1 ==
  note: $\delta(t)=tan^{-1} \left( \frac{2\ L\ sin(\alpha)}{l_{d}} \right)$
  alpha : Inport
  Atan : Trigonometry  Operator=atan
  Divide : Product  Inputs=*/
  Gain : Gain  Gain=2
  One over Look Ahead Distance : Constant  Value=lateral.lookAheadDistance
  Product : Product
  Sine Wave : Sin  TimeSource=Use external signal  SampleTime=0
  Wheel Base : Constant  Value=ego.wheelBase
  SteerCmd : Outport
  wires:
  Wheel Base/1 -> Gain/1
  Gain/1 -> Product/1
  Sine Wave/1 -> Product/2
  Product/1 -> Divide/1
  One over Look Ahead Distance/1 -> Divide/2
  Divide/1 -> Atan/1
  Atan/1 -> SteerCmd/1
  alpha/1 -> Sine Wave/1

== stateflow chart ManeuverPlanning/Unused Blocks/Driving Mode Selector ==
  state VehicleFollowing
    entry:
    drivingMode = 2;
  state FreeDrive
    entry:
    drivingMode = 1;
  state EmergecyBrake
    entry:
    drivingMode = 3;
  (default) -> FreeDrive
  VehicleFollowing -> FreeDrive [order 1] : [relativeDistance > 50]
  FreeDrive -> VehicleFollowing [order 1] : [relativeDistance <= 40]
  FreeDrive -> EmergecyBrake [order 2] : [relativeDistance <= 10]
  VehicleFollowing -> EmergecyBrake [order 2] : [relativeDistance <= 10]
  EmergecyBrake -> VehicleFollowing : [relativeDistance > 15]
  data: relativeDistance input; drivingMode output

== stateflow chart ManeuverPlanning/Unused Blocks/MPC/Driving Mode Selector ==
  state VehicleFollowing
    entry:
    drivingMode=2;
  state FreeDrive
    entry:
    drivingMode =1;
  state EmergecyBrake
    entry:
    drivingMode=3;
  (default) -> FreeDrive
  VehicleFollowing -> FreeDrive [order 1] : [relativeDistance >50]
  FreeDrive -> VehicleFollowing [order 1] : [relativeDistance <=40]
  FreeDrive -> EmergecyBrake [order 2] : [relativeDistance <=10]
  VehicleFollowing -> EmergecyBrake [order 2] : [relativeDistance <=10]
  EmergecyBrake -> VehicleFollowing : [relativeDistance>15]
  data: relativeDistance input; drivingMode output
